simulink model "gate"  (R2021b)
settings: Solver=VariableStepAuto  StartTime=0.0  StopTime=10.0  RelTol=1e-3
settings Model: Creator=soper  LastModifiedBy=soper

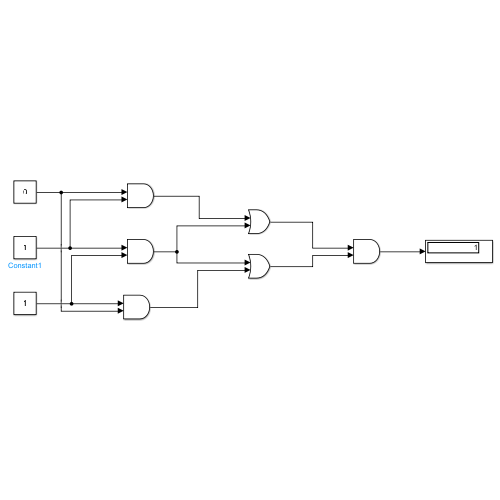
[thumbnail: Simulink's stored preview of the top-level diagram]
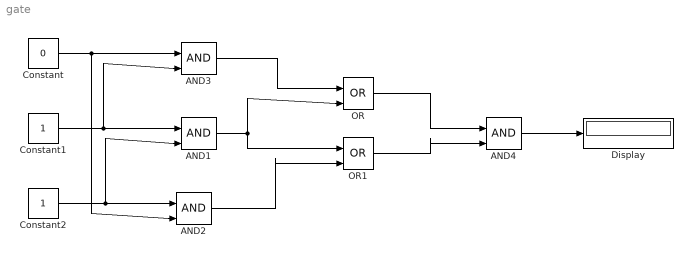
== system gate ==
  AND{1..4} (4 alike) : Logic  IconShape=distinctive  AllPortsSameDT=off  OutDataTypeStr=boolean
  Constant : Constant  Value=0
  Constant1 : Constant
  Constant2 : Constant
  Display : Display
  OR : Logic  Operator=OR  IconShape=distinctive  AllPortsSameDT=off  OutDataTypeStr=boolean
  OR1 : Logic  Operator=OR  IconShape=distinctive  AllPortsSameDT=off  OutDataTypeStr=boolean
  wires:
  Constant/1 -> AND2/2, AND3/1
  Constant1/1 -> AND3/2, AND1/1
  Constant2/1 -> AND1/2, AND2/1
  AND3/1 -> OR/1
  AND1/1 -> OR1/1, OR/2
  AND2/1 -> OR1/2
  OR/1 -> AND4/1
  OR1/1 -> AND4/2
  AND4/1 -> Display/1
